simulink model "UR5_OpenLoop"  (R2023b)
settings: Solver=FixedStepAuto  StartTime=0.0  StopTime=t_max  FixedStep=dt_max  RelTol=1e-3
values from neighbouring files (symbols this model uses):
  dt_max = 0.01    [UR5_Details.m]    (also in mpc_script.m; smc.m)
(part 1 of 2)
settings Model: Creator=sham_  LastModifiedBy=sham_

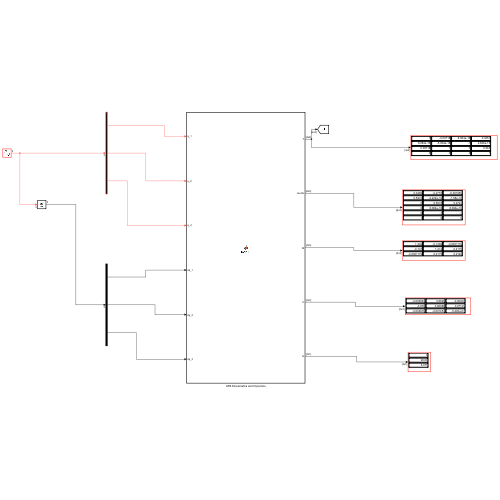
[thumbnail: Simulink's stored preview of the top-level diagram]
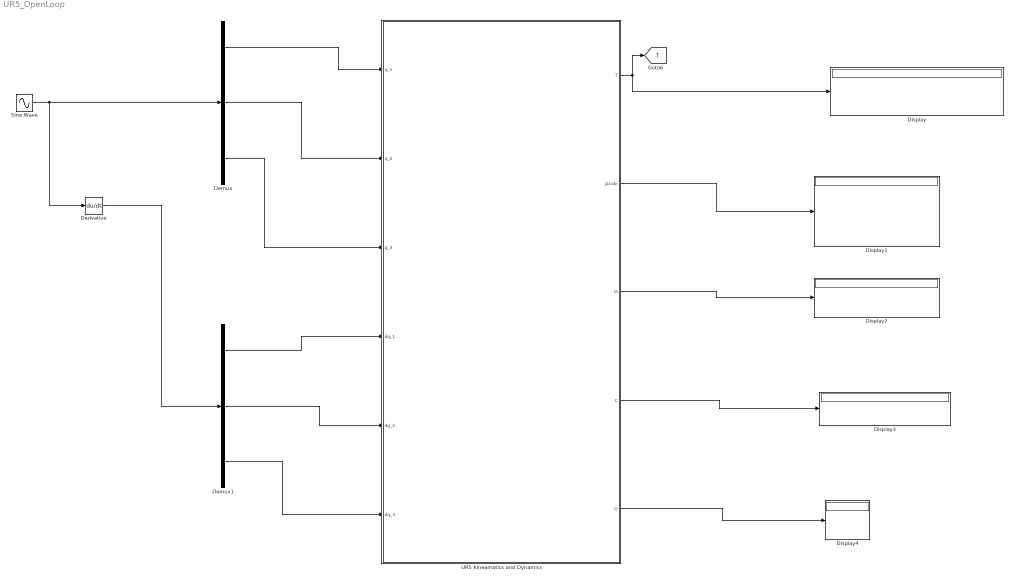
== system UR5_OpenLoop ==
  Demux : Demux  Outputs=3
  Demux1 : Demux  Outputs=3
  Derivative : Derivative
  Display{,1..4} (5 alike) : Display
  Sine Wave : Sin  Amplitude=[0.5, 0.7, 0.8]  Frequency=[pi,pi/2,pi/3]  SampleTime=dt_max
  UR5 Kineamatics and Dynamics : MATLAB Function  TreatAsAtomicUnit=on
  tag scope: T=global
  wires:
  UR5 Kineamatics and Dynamics/1(T) -> Display/1, [T]
  Demux/2 -> UR5 Kineamatics and Dynamics/2(q_2)
  Demux/1 -> UR5 Kineamatics and Dynamics/1(q_1)
  Demux/3 -> UR5 Kineamatics and Dynamics/3(q_3)
  UR5 Kineamatics and Dynamics/2(Jacobi) -> Display1/1
  UR5 Kineamatics and Dynamics/3(M) -> Display2/1
  UR5 Kineamatics and Dynamics/4(C) -> Display3/1
  UR5 Kineamatics and Dynamics/5(G) -> Display4/1
  Sine Wave/1 -> Derivative/1, Demux/1
  Demux1/1 -> UR5 Kineamatics and Dynamics/4(dq_1)
  Demux1/2 -> UR5 Kineamatics and Dynamics/5(dq_2)
  Demux1/3 -> UR5 Kineamatics and Dynamics/6(dq_3)
  Derivative/1 -> Demux1/1
